simulink model "mass_spring_model"  (R2014b)
settings: Solver=ode45  StartTime=0.0  StopTime=200  RelTol=1e-3
values from neighbouring files (symbols this model uses):
  B = 30    [mass_spring_force_data.mat]    (also in mass_spring_force_plot.m)
  F = 3000    [mass_spring_force_data.mat]    (also in mass_spring_force_plot.m = 30)
  K = 15    [mass_spring_force_data.mat]    (also in mass_spring_force_plot.m)
  M = 750    [mass_spring_force_data.mat]    (also in mass_spring_force_plot.m)
settings Model: Creator=Mashkoor Ahmed  LastModifiedBy=Mashkoor Ahmed

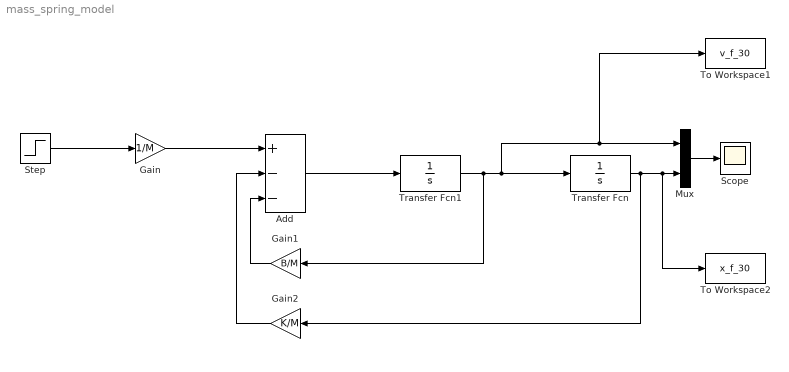
== system mass_spring_model ==
  Add : Sum  Inputs=+--
  Gain : Gain  Gain=1/M
  Gain1 : Gain  Gain=B/M
  Gain2 : Gain  Gain=K/M
  Mux : Mux  Inputs=2
  Scope : Scope
  Step : Step  Time=0  After=F  SampleTime=0
  To Workspace1 : ToWorkspace  VariableName=v_f_30  SaveFormat=Timeseries  SampleTime=-1
  To Workspace2 : ToWorkspace  VariableName=x_f_30  SaveFormat=Timeseries  SampleTime=-1
  Transfer Fcn : TransferFcn  Denominator=[1 0]
  Transfer Fcn1 : TransferFcn  Denominator=[1 0]
  wires:
  Step/1 -> Gain/1
  Gain/1 -> Add/1
  Gain1/1 -> Add/3
  Gain2/1 -> Add/2
  Add/1 -> Transfer Fcn1/1
  Transfer Fcn1/1 -> Gain1/1, To Workspace1/1, Mux/1, Transfer Fcn/1
  Transfer Fcn/1 -> Gain2/1, To Workspace2/1, Mux/2
  Mux/1 -> Scope/1
